simulink subsystem "INA219_Sensor"  (R2022b)
settings: Solver=VariableStepAuto  StartTime=0.0  StopTime=10.0  RelTol=1e-3
model mask{current_LSB=0.5, voltage_LSB=0.5, noise=on, i_noise_pwr=0, v_noise_pwr=0}
  mask prompts: current_LSB "Current quantization step:"; voltage_LSB "Voltage quantization step:"; noise "Simulate noise:"; i_noise_pwr "Current noise power:"; v_noise_pwr "Voltage noise power:"
libraries: simulink x2
settings Model: Creator=gotta  LastModifiedBy=gotta

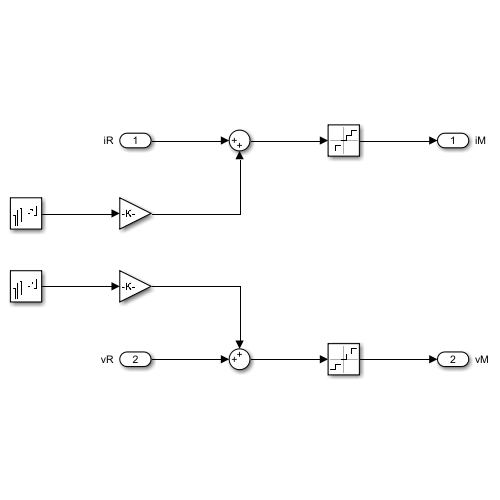
[thumbnail: Simulink's stored preview of the top-level diagram]
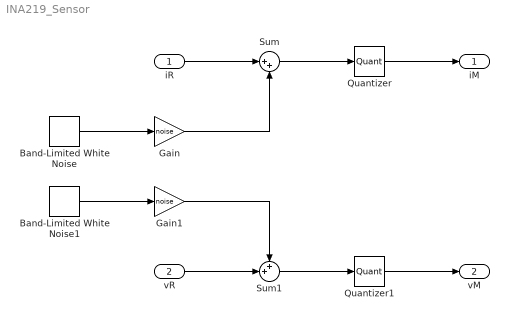
== system INA219_Sensor ==
  iR : Inport
  vR : Inport  Port=2
  Band-Limited White Noise : simulink/Sources/Band-Limited White Noise  Cov=i_noise_pwr  Ts=1e-3  seed=[23341]
  Band-Limited White Noise1 : simulink/Sources/Band-Limited White Noise  Cov=v_noise_pwr  Ts=1e-3  seed=[23341]
  Gain : Gain  Gain=noise  SampleTime=1e-3
  Gain1 : Gain  Gain=noise  SampleTime=1e-3
  Quantizer : Quantizer  QuantizationInterval=current_LSB
  Quantizer1 : Quantizer  QuantizationInterval=voltage_LSB
  Sum : Sum  Inputs=|++
  Sum1 : Sum  Inputs=++|
  iM : Outport
  vM : Outport  Port=2
  wires:
  Sum/1 -> Quantizer/1
  Sum1/1 -> Quantizer1/1
  Band-Limited White Noise/1 -> Gain/1
  Band-Limited White Noise1/1 -> Gain1/1
  Gain1/1 -> Sum1/1
  Gain/1 -> Sum/2
  iR/1 -> Sum/1
  vR/1 -> Sum1/2
  Quantizer/1 -> iM/1
  Quantizer1/1 -> vM/1
